simulink model "Heart3D_N43"  (R2024b)
settings: configuration reference "MasterConfig" (kept outside this file)
model workspace (MAT data in the model file):
  C_1 = 1
  C_10 = 23
  C_11 = 23
  C_12 = 23
  C_13 = 23
  C_14 = 23
  C_15 = 23
  C_16 = 23
  C_17 = 23
  C_18 = 23
  C_19 = 23
  C_2 = 1
  C_20 = 23
  C_21 = 23
  C_22 = 23
  C_23 = 2
  C_24 = 2
  C_25 = 2
  C_26 = 23
  C_27 = 23
  C_28 = 23
  C_29 = 23
  C_3 = 1
  C_30 = 50
  C_31 = 23
  C_32 = 23
  C_33 = 50
  C_34 = 23
  C_35 = 50
  C_36 = 23
  C_37 = 50
  C_38 = 50
  C_39 = 50
  C_4 = 1
  C_40 = 50
  C_41 = 50
  C_42 = 50
  C_43 = 50
  C_44 = 50
  C_45 = 23
  C_46 = 23
  C_47 = 23
  C_48 = 50
  C_49 = 50
  C_5 = 23
  C_50 = 23
  C_51 = 23
  C_52 = 23
  C_53 = 50
  C_54 = 50
  C_6 = 23
  C_7 = 23
  C_8 = 23
  C_9 = 23
  cfg : object (value not decoded)
  l_1 = 4.01400326634
  l_10 = 14.0362958077
  l_11 = 18.1950322891
  l_12 = 33.9599764429
  l_13 = 10
  l_14 = 8.0399004969
  l_15 = 12.0066648158
  l_16 = 7.69415362467
  l_17 = 5.21536192416
  l_18 = 5.65685424949
  l_19 = 13.8852439662
  l_2 = 3.2
  l_20 = 47.0387074652
  l_21 = 27.273430294
  l_22 = 13.8621787609
  l_23 = 18.6761880479
  l_24 = 12.8249756335
  l_25 = 15.879546593
  l_26 = 28.9689488936
  l_27 = 29.8073816361
  l_28 = 34.0352758179
  l_29 = 7.37563556583
  l_3 = 3.50907395191
  l_30 = 3.68781778292
  l_31 = 46.1042297409
  l_32 = 30.615028989
  l_33 = 7.51531769122
  l_34 = 7.47261667691
  l_35 = 3.73630833845
  l_36 = 36.7151195014
  l_37 = 16.1058995402
  l_38 = 48.7360236376
  l_39 = 48.8364617883
  l_4 = 4.54875807227
  l_40 = 41.4154560521
  l_41 = 37.7878287283
  l_42 = 44.689148571
  l_43 = 22.9120055866
  l_44 = 23.4401365184
  l_45 = 42.4264068712
  l_46 = 5
  l_47 = 8
  l_48 = 31.4273766007
  l_49 = 41.5788407727
  l_5 = 1.6986923075
  l_50 = 31.5569326773
  l_51 = 3
  l_52 = 3
  l_53 = 51.8478543433
  l_54 = 31.5569326773
  l_6 = 44.1540359298
  l_7 = 2.68208873828
  l_8 = 12.8
  l_9 = 4.53184289225
  xi_1 = 54.2
  xi_10 = 56.6
  xi_11 = 52.36
  xi_12 = 45
  xi_13 = 66.2
  xi_14 = 66.2
  xi_15 = 60.2
  xi_16 = 60.6
  xi_17 = 67
  xi_18 = 67.4
  xi_19 = 70.2
  xi_2 = 54.2
  xi_20 = 79.4
  xi_21 = 98.2
  xi_22 = 125.4
  xi_23 = 68.2
  xi_24 = 81.8
  xi_25 = 94.6
  xi_26 = 105
  xi_27 = 105
  xi_28 = 121.8
  xi_29 = 153
  xi_3 = 54.2
  xi_30 = 157.8
  xi_31 = 157.8
  xi_32 = 127.8
  xi_33 = 127.8
  xi_34 = 157
  xi_35 = 164.2
  xi_36 = 164.2
  xi_37 = 160.2
  xi_38 = 160.2
  xi_39 = 160.2
  xi_4 = 54.2
  xi_40 = 167.8
  xi_41 = 167.8
  xi_42 = 114.6
  xi_43 = 114.6
  xi_44 = 83
  xi_45 = 112.2
  xi_46 = 112.2
  xi_47 = 75
  xi_48 = 101.8
  xi_49 = 131
  xi_5 = 57.8666666667
  xi_50 = 159.4
  xi_51 = 159.4
  xi_52 = 143.4
  xi_53 = 112.2
  xi_54 = 162.4
  xi_6 = 57.8666666667
  xi_7 = 57.4
  xi_8 = 57.4
  xi_9 = 56.6
  xj_1 = 57.8666666667
  xj_10 = 66.2
  xj_11 = 45
  xj_12 = 53.8
  xj_13 = 60.2
  xj_14 = 67
  xj_15 = 60.6
  xj_16 = 68.2
  xj_17 = 67.4
  xj_18 = 68.2
  xj_19 = 79.4
  xj_2 = 57.4
  xj_20 = 118.6
  xj_21 = 125.4
  xj_22 = 135.4
  xj_23 = 81.8
  xj_24 = 94.6
  xj_25 = 105
  xj_26 = 121.8
  xj_27 = 127.8
  xj_28 = 153
  xj_29 = 157.8
  xj_3 = 56.6
  xj_30 = 160.2
  xj_31 = 112.2
  xj_32 = 157
  xj_33 = 131
  xj_34 = 164.2
  xj_35 = 167.8
  xj_36 = 159.4
  xj_37 = 167.8
  xj_38 = 114.6
  xj_39 = 112.2
  xj_4 = 52.36
  xj_40 = 131
  xj_41 = 162.4
  xj_42 = 83
  xj_43 = 131
  xj_44 = 101.8
  xj_45 = 75
  xj_46 = 112.2
  xj_47 = 67
  xj_48 = 125
  xj_49 = 101.8
  xj_5 = 57.4
  xj_50 = 143.4
  xj_51 = 162.4
  xj_52 = 146.4
  xj_53 = 67
  xj_54 = 146.4
  xj_6 = 98.2
  xj_7 = 56.6
  xj_8 = 70.2
  xj_9 = 52.36
  yi_1 = 118.2
  yi_10 = 115.64
  yi_11 = 114.04
  yi_12 = 97.4
  yi_13 = 105.4
  yi_14 = 105.4
  yi_15 = 97.4
  yi_16 = 85.4
  yi_17 = 97.4
  yi_18 = 92.2
  yi_19 = 118.2
  yi_2 = 118.2
  yi_20 = 107.8
  yi_21 = 137.8
  yi_22 = 139.8
  yi_23 = 86.6
  yi_24 = 99.4
  yi_25 = 100.2
  yi_26 = 88.2
  yi_27 = 88.2
  yi_28 = 64.6
  yi_29 = 51
  yi_3 = 118.2
  yi_30 = 45.4
  yi_31 = 45.4
  yi_32 = 69
  yi_33 = 69
  yi_34 = 59.8
  yi_35 = 57.8
  yi_36 = 57.8
  yi_37 = 42.6
  yi_38 = 42.6
  yi_39 = 42.6
  yi_4 = 118.2
  yi_40 = 56.8
  yi_41 = 56.8
  yi_42 = 59.8
  yi_43 = 59.8
  yi_44 = 91.4
  yi_45 = 38.6
  yi_46 = 38.6
  yi_47 = 59
  yi_48 = 105.4
  yi_49 = 75.8
  yi_5 = 119.833333333
  yi_50 = 94.2
  yi_51 = 94.2
  yi_52 = 121.4
  yi_53 = 33.6
  yi_54 = 94.2
  yi_6 = 119.833333333
  yi_7 = 118.2
  yi_8 = 118.2
  yi_9 = 115.64
  yj_1 = 119.833333333
  yj_10 = 105.4
  yj_11 = 97.4
  yj_12 = 64.6
  yj_13 = 97.4
  yj_14 = 97.4
  yj_15 = 85.4
  yj_16 = 86.6
  yj_17 = 92.2
  yj_18 = 86.6
  yj_19 = 107.8
  yj_2 = 118.2
  yj_20 = 133.8
  yj_21 = 139.8
  yj_22 = 130.2
  yj_23 = 99.4
  yj_24 = 100.2
  yj_25 = 88.2
  yj_26 = 64.6
  yj_27 = 69
  yj_28 = 51
  yj_29 = 45.4
  yj_3 = 115.64
  yj_30 = 42.6
  yj_31 = 38.6
  yj_32 = 59.8
  yj_33 = 75.8
  yj_34 = 57.8
  yj_35 = 56.8
  yj_36 = 94.2
  yj_37 = 56.8
  yj_38 = 59.8
  yj_39 = 33.6
  yj_4 = 114.04
  yj_40 = 75.8
  yj_41 = 94.2
  yj_42 = 91.4
  yj_43 = 75.8
  yj_44 = 105.4
  yj_45 = 59
  yj_46 = 33.6
  yj_47 = 59
  yj_48 = 126.6
  yj_49 = 105.4
  yj_5 = 118.2
  yj_50 = 121.4
  yj_51 = 94.2
  yj_52 = 121.4
  yj_53 = 59
  yj_54 = 121.4
  yj_6 = 137.8
  yj_7 = 115.64
  yj_8 = 118.2
  yj_9 = 114.04
  zi_1 = 0
  zi_10 = 0
  zi_11 = 0
  zi_12 = 0
  zi_13 = 0
  zi_14 = 0
  zi_15 = 0
  zi_16 = 0
  zi_17 = 0
  zi_18 = 0
  zi_19 = 0
  zi_2 = 0
  zi_20 = 0
  zi_21 = 0
  zi_22 = 0
  zi_23 = 0
  zi_24 = 0
  zi_25 = 0
  zi_26 = 0
  zi_27 = 0
  zi_28 = 0
  zi_29 = 0
  zi_3 = 0
  zi_30 = 0
  zi_31 = 0
  zi_32 = 0
  zi_33 = 0
  zi_34 = 0
  zi_35 = 0
  zi_36 = 0
  zi_37 = 0
  zi_38 = 0
  zi_39 = 0
  zi_4 = 0
  zi_40 = 0
  zi_41 = 0
  zi_42 = 0
  zi_43 = 0
  zi_44 = 0
  zi_45 = 0
  zi_46 = 0
  zi_47 = 0
  zi_48 = 0
  zi_49 = 0
  zi_5 = 0
  zi_50 = 0
  zi_51 = 0
  zi_52 = 0
  zi_53 = 0
  zi_54 = 0
  zi_6 = 0
  zi_7 = 0
  zi_8 = 0
  zi_9 = 0
  zj_1 = 0
  zj_10 = 0
  zj_11 = 0
  zj_12 = 0
  zj_13 = 0
  zj_14 = 0
  zj_15 = 0
  zj_16 = 0
  zj_17 = 0
  zj_18 = 0
  zj_19 = 0
  zj_2 = 0
  zj_20 = 0
  zj_21 = 0
  zj_22 = 0
  zj_23 = 0
  zj_24 = 0
  zj_25 = 0
  zj_26 = 0
  zj_27 = 0
  zj_28 = 0
  zj_29 = 0
  zj_3 = 0
  zj_30 = 0
  zj_31 = 0
  zj_32 = 0
  zj_33 = 0
  zj_34 = 0
  zj_35 = 0
  zj_36 = 0
  zj_37 = 0
  zj_38 = 0
  zj_39 = 0
  zj_4 = 0
  zj_40 = 0
  zj_41 = 0
  zj_42 = 0
  zj_43 = 0
  zj_44 = 0
  zj_45 = 0
  zj_46 = 0
  zj_47 = 0
  zj_48 = 0
  zj_49 = 0
  zj_5 = 0
  zj_50 = 0
  zj_51 = 0
  zj_52 = 0
  zj_53 = 0
  zj_54 = 0
  zj_6 = 0
  zj_7 = 0
  zj_8 = 0
  zj_9 = 0
symbols that are objects in the model workspace (value not decoded): cfg
(part 1 of 2)
settings Model: DataDictionary=Heart.sldd  EnableAccessToBaseWorkspace=off  Creator=wai484  LastModifiedBy=wai484
settings ConfigSetRef: SourceName=MasterConfig

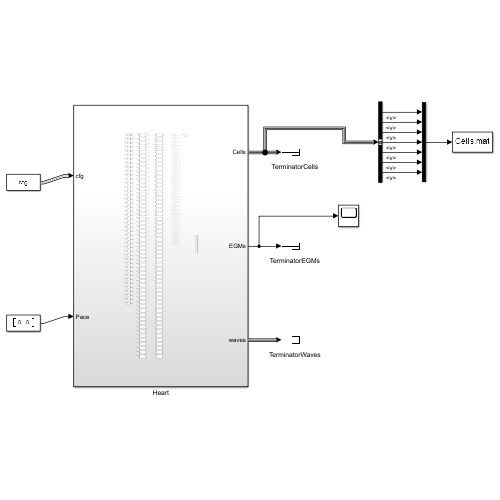
[thumbnail: Simulink's stored preview of the top-level diagram]
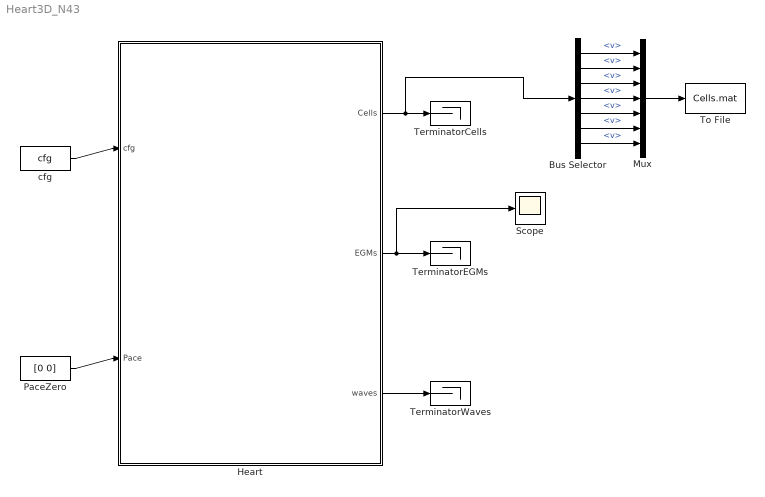
== system Heart3D_N43 ==
  Bus Selector : BusSelector  OutputSignals=c_SA.v,c_CT_a.v,c_RA.v,c_LA.v,c_LNB.v,c_LVm.v,c_RVm.v
  Heart : Subsystem
  Mux : Mux  Inputs=7
  PaceZero : Constant  Value=[0 0]
  Scope : Scope
  TerminatorCells : Terminator
  TerminatorEGMs : Terminator
  TerminatorWaves : Terminator
  To File : ToFile  Filename=Cells.mat  MatrixName=cell
      settings: Decimation=2
  cfg : Constant  Value=cfg  OutDataTypeStr=Bus: HeartCfgBus
  wires:
  Heart/1(Cells) -> Bus Selector/1, TerminatorCells/1
  Heart/2(EGMs) -> Scope/1, TerminatorEGMs/1
  Heart/3(waves) -> TerminatorWaves/1
  cfg/1 -> Heart/1(cfg)
  PaceZero/1 -> Heart/2(Pace)
  Bus Selector/1 -> Mux/1  "<v>"
  Bus Selector/2 -> Mux/2  "<v>"
  Bus Selector/3 -> Mux/3  "<v>"
  Bus Selector/4 -> Mux/4  "<v>"
  Bus Selector/5 -> Mux/5  "<v>"
  Bus Selector/6 -> Mux/6  "<v>"
  Bus Selector/7 -> Mux/7  "<v>"
  Mux/1 -> To File/1
